simulink subsystem "environment"  (R2025b)
settings: Solver=VariableStepAuto  StartTime=0.0  StopTime=10.0  RelTol=1e-3
undefined symbols (not defined in the file or in its folder): dt_env, Sim3dSensor
libraries: sim3dlib x5, sim3dcameralib x3
settings Model: Creator=koryh  LastModifiedBy=koryh

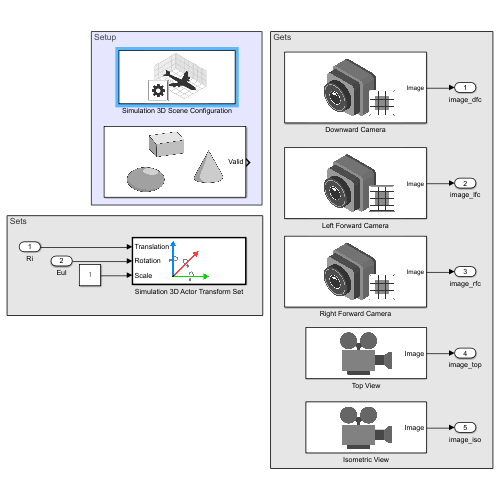
[thumbnail: Simulink's stored preview of the top-level diagram]
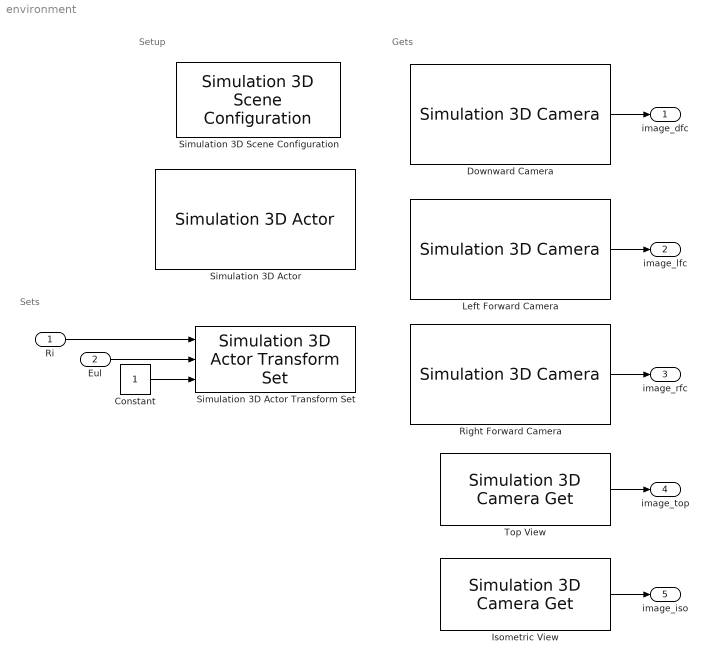
== system environment ==
  note: Sets
  note: Setup
  note: Gets
  Ri : Inport
  Eul : Inport  Port=2
  Constant : Constant
  Downward Camera : sim3dcameralib/Simulation 3D Camera  Priority=1  sensorTag=Sim3dSensor�  sensorId=1  sensorName=Sim3dSensor�  vehTagList={'Scene Origin';'Sim3dActor1'}  vehTag=Sim3dActor1  CoordinateSystem=ISO8855  mountLoc=Origin  offsetFlag=on  tmountOffset=[0, 0, 0]  extTmount=off  rmountOffset=[0, 0, 0]  extRmount=off  FocalLength=[1109, 1109]  OpticalCenter=[640, 360]  ImageSize=[720, 1280]  RadialDistortion=[0, 0]  TangentialDistortion=[0, 0]  SensorSkew=0  VisualizeFieldOfView=off  FieldOfViewRange=61  DepthOutportEnabled=off  SemanticOutportEnabled=off  TransformOutportEnabled=off  SampleTime=-1  mountPoint=[0 0 0]  mountOrientation=[0 0 0]  aMode=6  ID=1
      settings: LibrarySourceBlock=robotsim3dlib/Simulation 3D Camera
  Isometric View : sim3dlib/Simulation 3D Camera Get  Priority=1  sensorTag=Sim3dSensor�  sensorId=4  sensorName=Sim3dSensor�  vehTagList={'Scene Origin';'Sim3dActor1'}  vehTag=Sim3dActor1  CoordinateSystem=ISO8855  mountLoc=Origin  offsetFlag=off  tmountOffset=[0, 0, 0]  rmountOffset=[0, 0, 0]  HorizontalResolution=1280  VerticalResolution=720  HorizontalFOV=60  SampleTime=dt_env  mountPoint=[0 0 0]  mountOrientation=[0 0 0]  aMode=0  ID=4
      settings: LibrarySourceBlock=aerolibsim3d/Simulation 3D Camera Get
  Left Forward Camera : sim3dcameralib/Simulation 3D Camera  Priority=1  sensorTag=Sim3dSensor�  sensorId=2  sensorName=Sim3dSensor�  vehTagList={'Scene Origin';'Sim3dActor1'}  vehTag=Sim3dActor1  CoordinateSystem=ISO8855  mountLoc=Origin  offsetFlag=on  tmountOffset=[0, 0, 0]  extTmount=off  rmountOffset=[0, 0, 0]  extRmount=off  FocalLength=[1109, 1109]  OpticalCenter=[640, 360]  ImageSize=[720, 1280]  RadialDistortion=[0, 0]  TangentialDistortion=[0, 0]  SensorSkew=0  VisualizeFieldOfView=off  FieldOfViewRange=61  DepthOutportEnabled=off  SemanticOutportEnabled=off  TransformOutportEnabled=off  SampleTime=-1  mountPoint=[0 0 0]  mountOrientation=[0 0 0]  aMode=6  ID=2
      settings: LibrarySourceBlock=robotsim3dlib/Simulation 3D Camera
  Right Forward Camera : sim3dcameralib/Simulation 3D Camera  Priority=1  sensorTag=Sim3dSensor�  sensorId=3  sensorName=Sim3dSensor�  vehTagList={'Scene Origin';'Sim3dActor1'}  vehTag=Sim3dActor1  CoordinateSystem=ISO8855  mountLoc=Origin  offsetFlag=on  tmountOffset=[0, 0, 0]  extTmount=off  rmountOffset=[0, 0, 0]  extRmount=off  FocalLength=[1109, 1109]  OpticalCenter=[640, 360]  ImageSize=[720, 1280]  RadialDistortion=[0, 0]  TangentialDistortion=[0, 0]  SensorSkew=0  VisualizeFieldOfView=off  FieldOfViewRange=61  DepthOutportEnabled=off  SemanticOutportEnabled=off  TransformOutportEnabled=off  SampleTime=dt_env  mountPoint=[0 0 0]  mountOrientation=[0 0 0]  aMode=6  ID=3
      settings: LibrarySourceBlock=robotsim3dlib/Simulation 3D Camera
  Simulation 3D Actor : sim3dlib/Simulation 3D Actor  Priority=1  ActorName=Sim3dActor1  ParentName=Scene Origin  Operation=Create at setup  InitScriptText=|  SampleTime=-1  Translation=[0 0 0]  Rotation=[0 0 0]  Scale=[1 1 1]  aMode=5  ActorTag=Sim3dActor1  ActorType=Sim3dActor  ID=1
      | % Reserved keywords:
      | % - Actor : handle to this actor object
      | % - World : handle to the world object
      | 
      | % Examples:
      | 
      | % Create a primitive geometry (optional)
      | % createShape(Actor, 'box', [1 1 1]);
      | 
      | % Initialize values (optional)
      | % Actor.Physics = true;
      | % Actor.Color = [1 0 0];
  Simulation 3D Actor Transform Set : sim3dlib/Simulation 3D Actor Transform Set  Priority=-1  ActorTag=SimulinkActor1  CoordinateSystem=Default  NumberOfParts=1  CustNumOfParts=3  Translation=[0 0 0]  Rotation=[0 0 0]  Scale=[1 1 1]  Ts=-1  aMode=0
      settings: LibrarySourceBlock=aerolibsim3d/Simulation 3D Actor Transform Set
  Simulation 3D Scene Configuration : sim3dlib/Simulation 3D Scene Configuration  Priority=0  ProjectFormat=Unreal Editor  SceneDesc=Airport  ProjectName=C:\Program Files\MATLAB\R2025b\toolbox\shared\sim3d_projects\automotive_project_windows\UE\WindowsNoEditor\VehicleSimulation.exe  ScenePath=/Game/Maps/HwStrght  UEProjPath=C:\Users\koryh\Documents\Unreal Projects\MyProject2\MyProject2.uproject  EnableOpenDRIVE=off  vehTagList={'Custom';'Scene Origin';'Sim3dActor1'}  vehTag=Scene Origin  AttachedCameraRelativeTranslation=[0 0 0]  FreeCameraDefaultInitialTranslation=[-6, 0, 2]  AttachedCameraRelativeRotation=[0 0 0]  FreeCameraDefaultInitialRotation=[0, -15, 0]  ViewpointName=Custom  FreeCameraInitialTranslation=[-6, 0, 2]  ViewpointTranslation=[0 0 0]  FreeCameraInitialRotation=[0, -15, 0]  ViewpointRotation=[0 0 0]  OpVisEn=off  Ts=1/60  EnableWindow=on  EnableRemoteAccess=off  EnableWeather=off  SunAzimuth=90  SunAltitude=40.0  EnableGeospatialSun=off  Latitude=0  Longitude=0  Date=2023-01-01  Time=10:30:00  GeoTimeZone=-5.0  SunDaylightSaving=off  wind=1  clouds=10  EnableVolumetricClouds=off  CloudCoverage=0  CloudAltitude=6  fog=0  rain=0  RaindropsEffect=off  SnowDensity=0  EnableGeospatial=off  TilesetSource=Earth terrain  UseTrueOrigin=off  OriginHeight=200  OriginLatitude=40.744652  OriginLongitude=-73.988864  MapStyle=Aerial  AdditionalAssetIDs=[]  UseAdvancedSunSky=off  SolarTime=11  TimeZone=-5  Day=21  Month=9  Year=2022  UseDaylightSavingTime=on  DSTStartDay=10  DSTStartMonth=3  DSTEndDay=3  DSTEndMonth=11  DSTSwitchHour=2  sensorTag=MainCamera1  sensorId=1  sensorName=MainCamera1  mountLoc=Origin  offsetFlag=off  tmountOffset=[0, 0, 0]  rmountOffset=[0, 0, 0]  HorizontalResolution=1280  VerticalResolution=720  HorizontalFOV=60  mountPoint=[0 0 0]  mountOrientation=[0 0 0]  aMode=0  ID=1  GeoTrigger=Inactive  ViewNameList={'Custom'}  ViewTranslationList={'[-6 0 2]'}  ViewRotationList={'[0 -15 0]'}
      settings: LibrarySourceBlock=aerolibsim3d/Simulation 3D Scene Configuration
  Top View : sim3dlib/Simulation 3D Camera Get  Priority=1  sensorTag=Sim3dSensor�  sensorId=5  sensorName=Sim3dSensor�  vehTagList={'Scene Origin';'Sim3dActor1'}  vehTag=Sim3dActor1  CoordinateSystem=ISO8855  mountLoc=Origin  offsetFlag=off  tmountOffset=[0, 0, 0]  rmountOffset=[0, 0, 0]  HorizontalResolution=1280  VerticalResolution=720  HorizontalFOV=60  SampleTime=dt_env  mountPoint=[0 0 0]  mountOrientation=[0 0 0]  aMode=0  ID=5
      settings: LibrarySourceBlock=aerolibsim3d/Simulation 3D Camera Get
  image_dfc : Outport
  image_lfc : Outport  Port=2
  image_rfc : Outport  Port=3
  image_top : Outport  Port=4
  image_iso : Outport  Port=5
  wires:
  Top View/1 -> image_top/1
  Eul/1 -> Simulation 3D Actor Transform Set/2
  Ri/1 -> Simulation 3D Actor Transform Set/1
  Constant/1 -> Simulation 3D Actor Transform Set/3
  Right Forward Camera/1 -> image_rfc/1
  Downward Camera/1 -> image_dfc/1
  Left Forward Camera/1 -> image_lfc/1
  Isometric View/1 -> image_iso/1
